simulink subsystem "station1"  (R2024b)
settings: Solver=VariableStepAuto  StartTime=0.0  StopTime=10.0  RelTol=1e-3
undefined symbols (not defined in the file): DiscIntNeverNeededParam, DPL1ph, h, Half, R3, ResistanceM, Rt4, simetran, Ts, Zm
libraries: fl_lib x215, ee_lib x97, nesl_utility x43, spsThreePhaseHarmonicFilterLib x21, simulink x7, spsThreePhaseSeriesRLCLoadLib x7, spsThreePhaseBreakerLib x7
(part 6 of 6)

== system station1/Filters 60Hz7/tuned filter 11th ==
  Electrical Reference : fl_lib/Electrical/Electrical Elements/Electrical Reference
  Electrical Reference1 : fl_lib/Electrical/Electrical Elements/Electrical Reference
  Electrical Reference2 : fl_lib/Electrical/Electrical Elements/Electrical Reference
  Inductor : fl_lib/Electrical/Electrical Elements/Inductor  l=L1 H  r=R2 Ohm  g=1e-9 1/Ohm  i_specify=off  i_priority=None  i=0 A  i_nominal_specify=off  i_nominal_value=1  i_nominal_unit=A  v_specify=off  v_priority=None  v=0 V  v_nominal_specify=off  v_nominal_value=1  v_nominal_unit=V  i_L_specify=off  i_L_priority=High  i_L=0 A  i_L_nominal_specify=off  i_L_nominal_value=1  i_L_nominal_unit=A
  Inductor1 : fl_lib/Electrical/Electrical Elements/Inductor  l=L1 H  r=R2 Ohm  g=1e-9 1/Ohm  i_specify=off  i_priority=None  i=0 A  i_nominal_specify=off  i_nominal_value=1  i_nominal_unit=A  v_specify=off  v_priority=None  v=0 V  v_nominal_specify=off  v_nominal_value=1  v_nominal_unit=V  i_L_specify=off  i_L_priority=High  i_L=0 A  i_L_nominal_specify=off  i_L_nominal_value=1  i_L_nominal_unit=A
  Inductor2 : fl_lib/Electrical/Electrical Elements/Inductor  l=L1 H  r=R2 Ohm  g=1e-9 1/Ohm  i_specify=off  i_priority=None  i=0 A  i_nominal_specify=off  i_nominal_value=1  i_nominal_unit=A  v_specify=off  v_priority=None  v=0 V  v_nominal_specify=off  v_nominal_value=1  v_nominal_unit=V  i_L_specify=off  i_L_priority=High  i_L=0 A  i_L_nominal_specify=off  i_L_nominal_value=1  i_L_nominal_unit=A
  Phase Splitter : ee_lib/Connectors & References/Phase Splitter
  RC : fl_lib/Electrical/Electrical Elements/Capacitor  c=C1 F  r=0 Ohm  g=0 1/Ohm  i_specify=off  i_priority=None  i=0 A  i_nominal_specify=off  i_nominal_value=1  i_nominal_unit=A  v_specify=off  v_priority=None  v=0 V  v_nominal_specify=off  v_nominal_value=1  v_nominal_unit=V  vc_specify=off  vc_priority=High  vc=0 V  vc_nominal_specify=off  vc_nominal_value=1  vc_nominal_unit=V
  RC1 : fl_lib/Electrical/Electrical Elements/Capacitor  c=C1 F  r=0 Ohm  g=0 1/Ohm  i_specify=off  i_priority=None  i=0 A  i_nominal_specify=off  i_nominal_value=1  i_nominal_unit=A  v_specify=off  v_priority=None  v=0 V  v_nominal_specify=off  v_nominal_value=1  v_nominal_unit=V  vc_specify=off  vc_priority=High  vc=0 V  vc_nominal_specify=off  vc_nominal_value=1  vc_nominal_unit=V
  RC2 : fl_lib/Electrical/Electrical Elements/Capacitor  c=C1 F  r=0 Ohm  g=0 1/Ohm  i_specify=off  i_priority=None  i=0 A  i_nominal_specify=off  i_nominal_value=1  i_nominal_unit=A  v_specify=off  v_priority=None  v=0 V  v_nominal_specify=off  v_nominal_value=1  v_nominal_unit=V  vc_specify=off  vc_priority=High  vc=0 V  vc_nominal_specify=off  vc_nominal_value=1  vc_nominal_unit=V
  abc : PMIOPort  Side=Right
  connections:
  Inductor/LConn1 -- RC/RConn1
  Inductor/RConn1 -- Electrical Reference/LConn1
  RC1/RConn1 -- Inductor1/LConn1
  Inductor1/RConn1 -- Electrical Reference1/LConn1
  Inductor2/RConn1 -- Electrical Reference2/LConn1
  RC2/RConn1 -- Inductor2/LConn1
  Phase Splitter/RConn2 -- RC1/LConn1
  RC/LConn1 -- Phase Splitter/RConn1
  RC2/LConn1 -- Phase Splitter/RConn3
  Phase Splitter/LConn1 -- abc/RConn1

== system station1/Filters 60Hz7/tuned filter 13th ==
  Electrical Reference : fl_lib/Electrical/Electrical Elements/Electrical Reference
  Electrical Reference1 : fl_lib/Electrical/Electrical Elements/Electrical Reference
  Electrical Reference2 : fl_lib/Electrical/Electrical Elements/Electrical Reference
  Inductor : fl_lib/Electrical/Electrical Elements/Inductor  l=L1 H  r=R2 Ohm  g=1e-9 1/Ohm  i_specify=off  i_priority=None  i=0 A  i_nominal_specify=off  i_nominal_value=1  i_nominal_unit=A  v_specify=off  v_priority=None  v=0 V  v_nominal_specify=off  v_nominal_value=1  v_nominal_unit=V  i_L_specify=off  i_L_priority=High  i_L=0 A  i_L_nominal_specify=off  i_L_nominal_value=1  i_L_nominal_unit=A
  Inductor1 : fl_lib/Electrical/Electrical Elements/Inductor  l=L1 H  r=R2 Ohm  g=1e-9 1/Ohm  i_specify=off  i_priority=None  i=0 A  i_nominal_specify=off  i_nominal_value=1  i_nominal_unit=A  v_specify=off  v_priority=None  v=0 V  v_nominal_specify=off  v_nominal_value=1  v_nominal_unit=V  i_L_specify=off  i_L_priority=High  i_L=0 A  i_L_nominal_specify=off  i_L_nominal_value=1  i_L_nominal_unit=A
  Inductor2 : fl_lib/Electrical/Electrical Elements/Inductor  l=L1 H  r=R2 Ohm  g=1e-9 1/Ohm  i_specify=off  i_priority=None  i=0 A  i_nominal_specify=off  i_nominal_value=1  i_nominal_unit=A  v_specify=off  v_priority=None  v=0 V  v_nominal_specify=off  v_nominal_value=1  v_nominal_unit=V  i_L_specify=off  i_L_priority=High  i_L=0 A  i_L_nominal_specify=off  i_L_nominal_value=1  i_L_nominal_unit=A
  Phase Splitter : ee_lib/Connectors & References/Phase Splitter
  RC : fl_lib/Electrical/Electrical Elements/Capacitor  c=C1 F  r=0 Ohm  g=0 1/Ohm  i_specify=off  i_priority=None  i=0 A  i_nominal_specify=off  i_nominal_value=1  i_nominal_unit=A  v_specify=off  v_priority=None  v=0 V  v_nominal_specify=off  v_nominal_value=1  v_nominal_unit=V  vc_specify=off  vc_priority=High  vc=0 V  vc_nominal_specify=off  vc_nominal_value=1  vc_nominal_unit=V
  RC1 : fl_lib/Electrical/Electrical Elements/Capacitor  c=C1 F  r=0 Ohm  g=0 1/Ohm  i_specify=off  i_priority=None  i=0 A  i_nominal_specify=off  i_nominal_value=1  i_nominal_unit=A  v_specify=off  v_priority=None  v=0 V  v_nominal_specify=off  v_nominal_value=1  v_nominal_unit=V  vc_specify=off  vc_priority=High  vc=0 V  vc_nominal_specify=off  vc_nominal_value=1  vc_nominal_unit=V
  RC2 : fl_lib/Electrical/Electrical Elements/Capacitor  c=C1 F  r=0 Ohm  g=0 1/Ohm  i_specify=off  i_priority=None  i=0 A  i_nominal_specify=off  i_nominal_value=1  i_nominal_unit=A  v_specify=off  v_priority=None  v=0 V  v_nominal_specify=off  v_nominal_value=1  v_nominal_unit=V  vc_specify=off  vc_priority=High  vc=0 V  vc_nominal_specify=off  vc_nominal_value=1  vc_nominal_unit=V
  abc : PMIOPort  Side=Right
  connections:
  Phase Splitter/LConn1 -- abc/RConn1
  RC2/LConn1 -- Phase Splitter/RConn3
  RC/LConn1 -- Phase Splitter/RConn1
  Phase Splitter/RConn2 -- RC1/LConn1
  RC2/RConn1 -- Inductor2/LConn1
  Inductor2/RConn1 -- Electrical Reference2/LConn1
  Inductor1/RConn1 -- Electrical Reference1/LConn1
  RC1/RConn1 -- Inductor1/LConn1
  Inductor/RConn1 -- Electrical Reference/LConn1
  Inductor/LConn1 -- RC/RConn1

== system station1/Half-DPL1ph/Simscape ==
  Electrical Reference1 : fl_lib/Electrical/Electrical Elements/Electrical Reference
  PS-S : nesl_utility/PS-Simulink Converter  PhysicalDomain=network_engine_domain  SubClassName=ps_output  LeftPortType=input  RightPortType=output  PseudoPeriodic=off  Frequencies=[]  VectorFormat=1-D array  Unit=V  AffineConversion=off
  Voltage Sensor : fl_lib/Electrical/Electrical Sensors/Voltage Sensor
  V : PMIOPort  Side=Left
  Out : Outport  VectorParamsAs1DForOutWhenUnconnected=off
  wires:
  PS-S/1 -> Out/1  "voltage"
  connections:
  PS-S/LConn1 -- Voltage Sensor/RConn1
  V/RConn1 -- Voltage Sensor/LConn1
  Electrical Reference1/LConn1 -- Voltage Sensor/RConn2

== system station1/Half-DPL1ph/Voltage Source ==
  I : Inport
  Controlled Current Source1 : fl_lib/Electrical/Electrical Sources/Controlled Current Source
  Simulink-PS Converter : nesl_utility/Simulink-PS Converter  PhysicalDomain=network_engine_domain  SubClassName=ps_input  LeftPortType=input  RightPortType=output  PseudoPeriodic=off  Frequencies=[]  NoiseDistribution=none  NoiseParameters=[]  Unit=1  AffineConversion=off  FilteringAndDerivatives=zero  SimscapeFilterOrder=1  InputFilterTimeConstant=.001  UdotUserProvided=0
  + : PMIOPort  Side=Right
  - : PMIOPort  Port=2  Side=Right
  wires:
  I/1 -> Simulink-PS Converter/1
  connections:
  Controlled Current Source1/RConn1 -- Simulink-PS Converter/RConn1
  Controlled Current Source1/RConn2 -- -/RConn1
  Controlled Current Source1/LConn1 -- +/RConn1

== system station1/Half-DPL1ph/dplmodel ==
  v : Inport
  hist_in : Inport  Port=2
  (1+h)/Z : Gain  Gain=(1+h)./(Zm+Rt4)  SaturateOnIntegerOverflow=on  OutDataTypeStr=Inherit: Same as input  ParamDataTypeStr=Inherit: Same as input
  Gain4 : Gain  Gain=(1+h)/2  SaturateOnIntegerOverflow=on  OutDataTypeStr=Inherit: Same as input  ParamDataTypeStr=Inherit: Same as input
  Gain6 : Gain  Gain=(1-h)/2  SaturateOnIntegerOverflow=on  OutDataTypeStr=Inherit: Same as input  ParamDataTypeStr=Inherit: Same as input
  Gain9 : Gain  Gain=h  SaturateOnIntegerOverflow=on  OutDataTypeStr=Inherit: Same as input  ParamDataTypeStr=Inherit: Same as input
  Sum1 : Sum  Inputs=-+  InputSameDT=on  SaturateOnIntegerOverflow=on  OutDataTypeStr=Inherit: Same as first input
  Sum3 : Sum  InputSameDT=on  SaturateOnIntegerOverflow=on  OutDataTypeStr=Inherit: Same as first input
  derlay : Subsystem
  i : Outport  InitialOutput=0  VectorParamsAs1DForOutWhenUnconnected=off
  hist_out : Outport  Port=2  VectorParamsAs1DForOutWhenUnconnected=off
  wires:
  Sum3/1 -> i/1, Gain9/1
  v/1 -> (1+h)/Z/1
  Gain4/1 -> hist_out/1
  Gain9/1 -> Sum1/1
  (1+h)/Z/1 -> Sum1/2
  Gain6/1 -> Sum3/1
  hist_in/1 -> Sum3/2
  derlay/1(Out1) -> Gain4/1, Gain6/1
  Sum1/1 -> derlay/1(In1)

== system station1/Half-DPL1ph1/Simscape ==
  Electrical Reference1 : fl_lib/Electrical/Electrical Elements/Electrical Reference
  PS-S : nesl_utility/PS-Simulink Converter  PhysicalDomain=network_engine_domain  SubClassName=ps_output  LeftPortType=input  RightPortType=output  PseudoPeriodic=off  Frequencies=[]  VectorFormat=1-D array  Unit=V  AffineConversion=off
  Voltage Sensor : fl_lib/Electrical/Electrical Sensors/Voltage Sensor
  V : PMIOPort  Side=Left
  Out : Outport  VectorParamsAs1DForOutWhenUnconnected=off
  wires:
  PS-S/1 -> Out/1  "voltage"
  connections:
  Electrical Reference1/LConn1 -- Voltage Sensor/RConn2
  V/RConn1 -- Voltage Sensor/LConn1
  PS-S/LConn1 -- Voltage Sensor/RConn1

== system station1/Half-DPL1ph1/Voltage Source ==
  I : Inport
  Controlled Current Source1 : fl_lib/Electrical/Electrical Sources/Controlled Current Source
  Simulink-PS Converter : nesl_utility/Simulink-PS Converter  PhysicalDomain=network_engine_domain  SubClassName=ps_input  LeftPortType=input  RightPortType=output  PseudoPeriodic=off  Frequencies=[]  NoiseDistribution=none  NoiseParameters=[]  Unit=1  AffineConversion=off  FilteringAndDerivatives=zero  SimscapeFilterOrder=1  InputFilterTimeConstant=.001  UdotUserProvided=0
  + : PMIOPort  Side=Right
  - : PMIOPort  Port=2  Side=Right
  wires:
  I/1 -> Simulink-PS Converter/1
  connections:
  Controlled Current Source1/LConn1 -- +/RConn1
  Controlled Current Source1/RConn2 -- -/RConn1
  Controlled Current Source1/RConn1 -- Simulink-PS Converter/RConn1

== system station1/Half-DPL1ph1/dplmodel ==
  v : Inport
  hist_in : Inport  Port=2
  (1+h)/Z : Gain  Gain=(1+h)./(Zm+Rt4)  SaturateOnIntegerOverflow=on  OutDataTypeStr=Inherit: Same as input  ParamDataTypeStr=Inherit: Same as input
  Gain4 : Gain  Gain=(1+h)/2  SaturateOnIntegerOverflow=on  OutDataTypeStr=Inherit: Same as input  ParamDataTypeStr=Inherit: Same as input
  Gain6 : Gain  Gain=(1-h)/2  SaturateOnIntegerOverflow=on  OutDataTypeStr=Inherit: Same as input  ParamDataTypeStr=Inherit: Same as input
  Gain9 : Gain  Gain=h  SaturateOnIntegerOverflow=on  OutDataTypeStr=Inherit: Same as input  ParamDataTypeStr=Inherit: Same as input
  Sum1 : Sum  Inputs=-+  InputSameDT=on  SaturateOnIntegerOverflow=on  OutDataTypeStr=Inherit: Same as first input
  Sum3 : Sum  InputSameDT=on  SaturateOnIntegerOverflow=on  OutDataTypeStr=Inherit: Same as first input
  derlay : Subsystem
  i : Outport  InitialOutput=0  VectorParamsAs1DForOutWhenUnconnected=off
  hist_out : Outport  Port=2  VectorParamsAs1DForOutWhenUnconnected=off
  wires:
  Sum1/1 -> derlay/1(In1)
  derlay/1(Out1) -> Gain6/1, Gain4/1
  hist_in/1 -> Sum3/2
  Gain6/1 -> Sum3/1
  (1+h)/Z/1 -> Sum1/2
  Gain9/1 -> Sum1/1
  Gain4/1 -> hist_out/1
  v/1 -> (1+h)/Z/1
  Sum3/1 -> Gain9/1, i/1

== system station1/Half-DPL1ph/dplmodel/derlay ==
  In1 : Inport
  Add : Sum
  Delay1 : Delay  DelayLength=delay(1)
  Gain : Gain  Gain=remd
  Gain1 : Gain  Gain=1-remd
  Unit Delay1 : UnitDelay  SampleTime=Ts  HasFrameUpgradeWarning=on
  Out1 : Outport
  wires:
  In1/1 -> Delay1/1
  Gain/1 -> Add/1
  Gain1/1 -> Add/2
  Unit Delay1/1 -> Gain/1
  Add/1 -> Out1/1
  Delay1/1 -> Gain1/1, Unit Delay1/1

== system station1/Half-DPL1ph1/dplmodel/derlay ==
  In1 : Inport
  Add : Sum
  Delay1 : Delay  DelayLength=delay(1)
  Gain : Gain  Gain=remd
  Gain1 : Gain  Gain=1-remd
  Unit Delay1 : UnitDelay  SampleTime=Ts  HasFrameUpgradeWarning=on
  Out1 : Outport
  wires:
  Delay1/1 -> Unit Delay1/1, Gain1/1
  Add/1 -> Out1/1
  Unit Delay1/1 -> Gain/1
  Gain1/1 -> Add/2
  Gain/1 -> Add/1
  In1/1 -> Delay1/1
